simulink model "ledblink"  (R2023a)
settings: Solver=VariableStepAuto  StartTime=0.0  StopTime=10.0  RelTol=1e-3
settings Model: Creator=Egypt_Laptop  LastModifiedBy=Egypt_Laptop

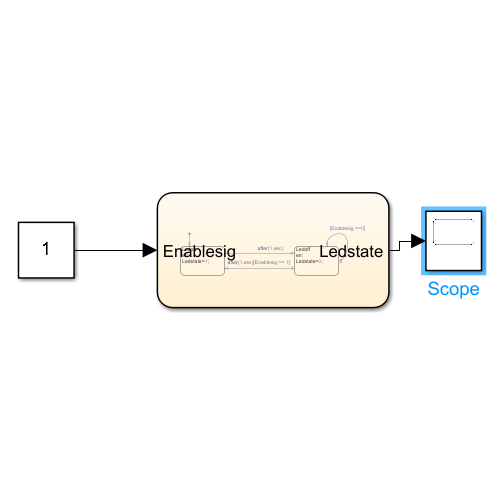
[thumbnail: Simulink's stored preview of the top-level diagram]
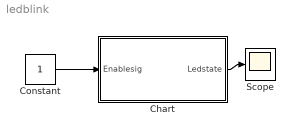
== system ledblink ==
  Chart : Stateflow chart  TreatAsAtomicUnit=on
  Constant : Constant
  Scope : Scope
  wires:
  Chart/1(Ledstate) -> Scope/1
  Constant/1 -> Chart/1(Enablesig)

== stateflow chart ledblink/Chart ==
  state Ledon
    en:
    Ledstate=1;
  state Ledoff
    en:
    Ledstate=0;
  (default) -> Ledon
  Ledoff -> Ledoff [order 2] : [Enablesig ==0]
  Ledon -> Ledoff : after(1,sec)
  Ledoff -> Ledon [order 1] : after(1,sec)[Enablesig == 1]
  data: Ledstate output double; Enablesig input double
